simulink model "Model14"  (R2020a)
settings: Solver=VariableStepAuto  StartTime=0.0  StopTime=70  RelTol=1e-3
values from neighbouring files (symbols this model uses):
  Cf = 100000    [Model12_MATscript.m]
  Cr = 110000    [Model12_MATscript.m]
undefined symbols (not defined in the file or in its folder): a, a0, a1, a10, a11, a12, a13, a14, a15, a16, a17, a2, a3, a4, a5, a6, a7, a8, a9, alpha, Area, b, b1, b11, b12, b2, banking_indy, bankingON, C_fuel, camber, curveCenters, Cx, Cz, distanceThreshold, g, init_vel, init_x_pos, init_y_pos, init_yaw, IT, K_wear, l_f, l_r, longStraight, lookahead, m_fuel, mT, overlapThreshold, radius_second_lane, rho_0, rho_1, shortStraight, slipstreamON, trajec, turn, TyreContactAreaFront, TyreContactAreaRear, w1, w2
libraries: simulink x5
(part 1 of 2)
settings Model: PacingRate=2  Creator=carmelo  LastModifiedBy=cvalo

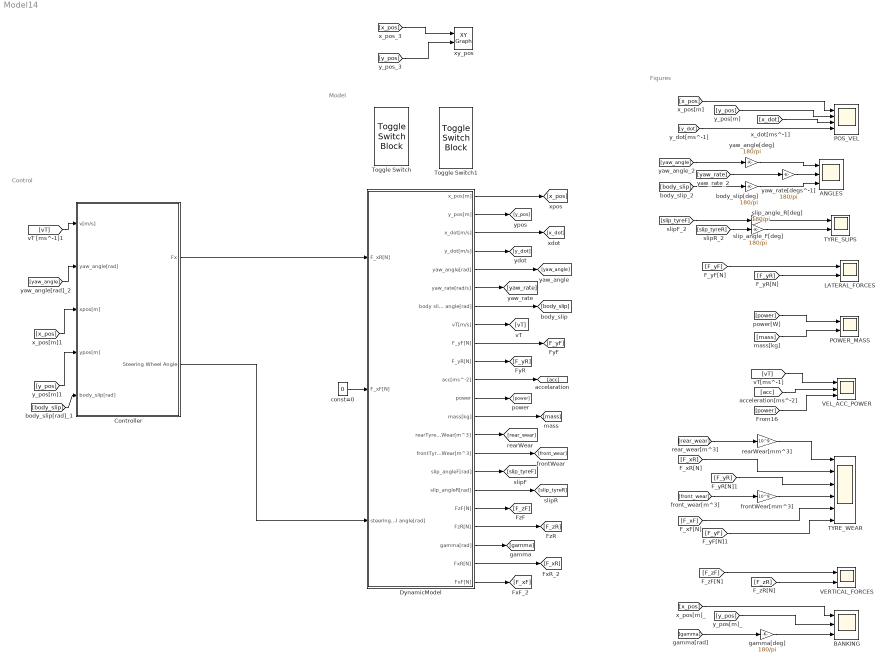
== system Model14 ==
  note: Control
  note: Model
  note: Figures
  ANGLES : Scope  NumInputPorts=3
  BANKING : Scope  NumInputPorts=3
  Controller : Subsystem
  DynamicModel : Subsystem
  LATERAL_FORCES : Scope  NumInputPorts=2
  POS_VEL : Scope  NumInputPorts=4
  POWER_MASS : Scope  NumInputPorts=2
  TYRE_SLIPS : Scope  NumInputPorts=2
  TYRE_WEAR : Scope  NumInputPorts=6
  Toggle Switch : ToggleSwitchBlock
      settings: Values={{'Off', 'On'}, [0 1]}
  Toggle Switch1 : ToggleSwitchBlock
      settings: Values={{'Off', 'On'}, [0 1]}
  VEL_ACC_POWER : Scope  NumInputPorts=3
  VERTICAL_FORCES : Scope  NumInputPorts=2
  body_slip[deg] : Gain  Gain=180/pi
  const=0 : Constant  Value=0
  frontWear[mm^3] : Gain  Gain=10^9
  gamma[deg] : Gain  Gain=180/pi
  rearWear[mm^3] : Gain  Gain=10^9
  slip_angle_F[deg] : Gain  Gain=180/pi
  slip_angle_R[deg] : Gain  Gain=180/pi
  xy_pos : simulink/Sinks/XY Graph  xmin=-900  xmax=900  ymin=-50  ymax=800  st=-1
  yaw_angle[deg] : Gain  Gain=180/pi
  yaw_rate[degs^-1] : Gain  Gain=180/pi
  wires:
  DynamicModel/3(x_dot[m/s]) -> [x_dot]
  DynamicModel/4(y_dot[m/s]) -> [y_dot]
  DynamicModel/1(x_pos[m]) -> [x_pos]
  DynamicModel/2(y_pos[m]) -> [y_pos]
  Controller/2(Steering Wheel Angle) -> DynamicModel/3(steering wheel angle[rad])
  DynamicModel/5(yaw_angle[rad]) -> [yaw_angle]
  DynamicModel/6(yaw_rate[rad/s]) -> [yaw_rate]
  DynamicModel/7(body slip angle[rad]) -> [body_slip]
  DynamicModel/8(vT[m/s]) -> [vT]
  DynamicModel/9(F_yF[N]) -> [F_yF]
  DynamicModel/10(F_yR[N]) -> [F_yR]
  DynamicModel/11(acc[ms^-2]) -> [acc]
  DynamicModel/12(power) -> [power]
  DynamicModel/13(mass[kg]) -> [mass]
  DynamicModel/15(frontTyreWear[m^3]) -> [front_wear]
  DynamicModel/14(rearTyreWear[m^3]) -> [rear_wear]
  DynamicModel/16(slip_angleF[rad]) -> [slip_tyreF]
  DynamicModel/17(slip_angleR[rad]) -> [slip_tyreR]
  slip_angle_R[deg]/1 -> TYRE_SLIPS/2
  [x_pos] -> POS_VEL/1
  [front_wear] -> frontWear[mm^3]/1
  [mass] -> POWER_MASS/2
  yaw_rate[degs^-1]/1 -> ANGLES/2
  body_slip[deg]/1 -> ANGLES/3
  [yaw_angle] -> yaw_angle[deg]/1
  [y_dot] -> POS_VEL/4
  [y_pos] -> POS_VEL/2
  [yaw_rate] -> yaw_rate[degs^-1]/1
  [body_slip] -> body_slip[deg]/1
  [power] -> POWER_MASS/1
  [acc] -> VEL_ACC_POWER/2
  [rear_wear] -> rearWear[mm^3]/1
  yaw_angle[deg]/1 -> ANGLES/1
  [F_yR] -> LATERAL_FORCES/2
  [slip_tyreR] -> slip_angle_R[deg]/1
  [slip_tyreF] -> slip_angle_F[deg]/1
  [F_yF] -> LATERAL_FORCES/1
  [power] -> VEL_ACC_POWER/3
  [x_dot] -> POS_VEL/3
  slip_angle_F[deg]/1 -> TYRE_SLIPS/1
  [vT] -> VEL_ACC_POWER/1
  rearWear[mm^3]/1 -> TYRE_WEAR/1
  frontWear[mm^3]/1 -> TYRE_WEAR/4
  [x_pos] -> xy_pos/1
  [y_pos] -> xy_pos/2
  const=0/1 -> DynamicModel/2(F_xF[N])
  Controller/1(Fx) -> DynamicModel/1(F_xR[N])
  [F_xF] -> TYRE_WEAR/5
  [F_yF] -> TYRE_WEAR/6
  [F_xR] -> TYRE_WEAR/2
  [F_yR] -> TYRE_WEAR/3
  [vT] -> Controller/1(v[m/s])
  DynamicModel/18(FzF[N]) -> [F_zF]
  DynamicModel/19(FzR[N]) -> [F_zR]
  DynamicModel/20(gamma[rad]) -> [gamma]
  [F_zF] -> VERTICAL_FORCES/1
  [F_zR] -> VERTICAL_FORCES/2
  [y_pos] -> BANKING/2
  [x_pos] -> BANKING/1
  [gamma] -> gamma[deg]/1
  gamma[deg]/1 -> BANKING/3
  [yaw_angle] -> Controller/2(yaw_angle[rad])
  [y_pos] -> Controller/4(ypos[m])
  [x_pos] -> Controller/3(xpos[m])
  DynamicModel/21(FxR[N]) -> [F_xR]
  DynamicModel/22(FxF[N]) -> [F_xF]
  [body_slip] -> Controller/5(body_slip[rad])

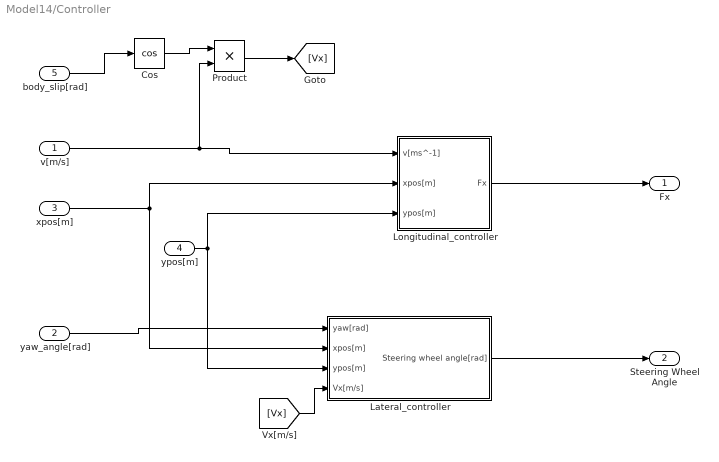
== system Model14/Controller ==
  v[m/s] : Inport  Unit=m/s
  yaw_angle[rad] : Inport  Port=2
  xpos[m] : Inport  Port=3
  ypos[m] : Inport  Port=4
  body_slip[rad] : Inport  Port=5
  Cos : Trigonometry  Operator=cos
  Lateral_controller : Subsystem
  Longitudinal_controller : Subsystem
  Product : Product
  Fx : Outport  Unit=N
  Steering Wheel Angle : Outport  Port=2  Unit=rad
  wires:
  Lateral_controller/1(Steering wheel angle[rad]) -> Steering Wheel Angle/1
  v[m/s]/1 -> Product/2, Longitudinal_controller/1(v[ms^-1])
  yaw_angle[rad]/1 -> Lateral_controller/1(yaw[rad])
  xpos[m]/1 -> Lateral_controller/2(xpos[m]), Longitudinal_controller/2(xpos[m])
  ypos[m]/1 -> Lateral_controller/3(ypos[m]), Longitudinal_controller/3(ypos[m])
  Longitudinal_controller/1(Fx) -> Fx/1
  body_slip[rad]/1 -> Cos/1
  Cos/1 -> Product/1
  Product/1 -> [Vx]
  [Vx] -> Lateral_controller/4(Vx[m/s])

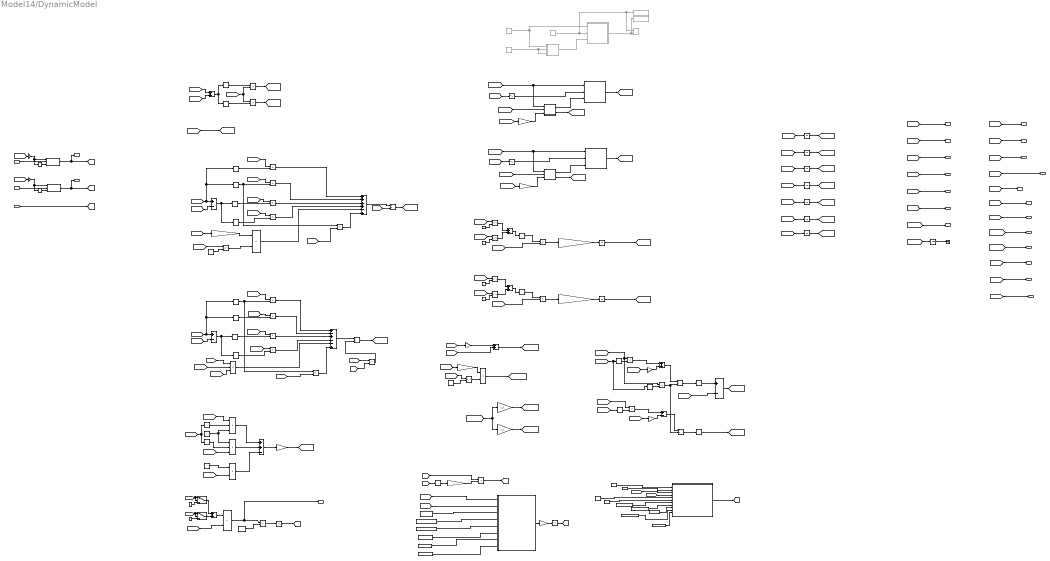
== system Model14/DynamicModel ==
  note: Inputs
  note: Wind effect
  note: FN
  note: Tyre wears
  note: Outputs
  note: Tires slip angles
  note: Tire lateral forces
  note: x6_dot equation
  note: Continuos integration
  note: x4_dot equation
  note: x3_dot equation
  note: x1_dot and x2_dot equations
  note: x5_dot equation
  note: mdot
  note: vertical force
  F_xR[N] : Inport  Unit=N
  F_xF[N] : Inport  Port=2  Unit=N
  steering wheel angle[rad] : Inport  Port=3  Unit=rad
  (F_xR+F_xF)*vT : Product
  (F_xR+F_xF)*vT*c_fuel : Product
  -FxmaxF : UnaryMinus
  -FxmaxR : UnaryMinus
  -b*x6+vT*sin(x5) : Sum  Inputs=+-
  -banking : UnaryMinus
  -slip_angle_F : UnaryMinus
  -slip_angle_R : UnaryMinus
  Banking : MATLAB Function  TreatAsAtomicUnit=on
  BankingON-OFF : Constant  Value=bankingON
  Calculate Peak F : Subsystem
  Calculate Peak F1 : Subsystem  Commented=on
  Calculate Peak R : Subsystem
  Constant : Constant  Value=banking_indy
  FNx*cos(x5) : Product
  FNx*sin(x5) : Product
  FNx_4 : Product
  F_aerod : Product
  F_lift_3 : Product
  F_xF*cos(x5-delta) : Product
  F_xF*sin(x5-delta) : Product
  F_xR*cos(x5) : Product
  F_xR*sin(x5) : Product
  F_xR+F_xF : Sum
  F_yF*cos(x5-delta) : Product
  F_yF*sin(x5-delta) : Product
  F_yR*cos(x5) : Product
  F_yR*sin(x5) : Product
  FrontWearDot : Gain  Gain=K_wear/TyreContactAreaFront
  FrontWearIntegrator : Integrator
  Front_Wear*10^9 : Gain  Gain=10^9
  FxF^2 : Math  Operator=pow  SaturateOnIntegerOverflow=on
  FxF^2+FyF^2 : Sum
  FxR^2 : Math  Operator=pow  SaturateOnIntegerOverflow=on
  FxR^2+FyR^2 : Sum
  FyF^2 : Math  Operator=pow  SaturateOnIntegerOverflow=on
  FyR^2 : Math  Operator=pow  SaturateOnIntegerOverflow=on
  Fz*lf : Gain  Gain=l_f
  Fz*lr : Gain  Gain=l_r
  FzF*sqrt(FxF^2+FyF^2) : Product
  FzR*sqrt(FxR^2+FyR^2) : Product
  PacejkaF : Subsystem
  PacejkaF1 : Subsystem  Commented=on
  PacejkaR : Subsystem
  RearWearDot : Gain  Gain=K_wear/TyreContactAreaRear
  RearWearIntegrator : Integrator
  Rear_Wear*10^9 : Gain  Gain=10^9
  Saturation Dynamic : simulink/Discontinuities/Saturation Dynamic  OutMin=[]  OutMax=[]  OutDataTypeStr=Inherit: Same as second input  OutDataType=fixdt(1, 16)  OutScaling=2^-10  DoSatur=off
  Saturation Dynamic1 : simulink/Discontinuities/Saturation Dynamic  OutMin=[]  OutMax=[]  OutDataTypeStr=Inherit: Same as second input  OutDataType=fixdt(1, 16)  OutScaling=2^-10  DoSatur=off
  Terminator : Terminator
  To Workspace : ToWorkspace  Commented=on  VariableName=alfaPaj  SaveFormat=Timeseries  SampleTime=-1
  To Workspace1 : ToWorkspace  Commented=on  VariableName=FyPaj  SaveFormat=Timeseries  SampleTime=-1
  WindEffect : MATLAB Function  TreatAsAtomicUnit=on
  XY Graph : simulink/Sinks/XY Graph  Commented=on  xmin=-1  xmax=1  ymin=-8500  ymax=8500  st=-1
  a*F_xF*sin(delta) : Product  Inputs=3
  a*F_xF*sin(delta)+ a*F_yF*cos(delta)+ b*F_yR : Sum  Inputs=++-
  a*F_yF*cos(delta) : Product  Inputs=3
  a*x6 : Gain  Gain=a
  a*x6+vT*sin(x5) : Sum
  a*x6+vT*sin(x5) -------------------- vT*cos(x5) : Product  Inputs=*/
  alpha : Constant  Value=alpha
  alpha-1+1 : simulink/Sources/Ramp  Commented=on  slope=0.02  start=0  InitialOutput=-1
  atan(-b*x6+vT*sin(x5) -------------------- vT*cos(x5)) : Trigonometry  Operator=atan
  atan(a*x6+vT*sin(x5) -------------------- vT*cos(x5)) : Trigonometry  Operator=atan
  b*F_yR : Product
  b*x6 : Gain  Gain=b
  b*x6+vT*sin(x5) -------------------- vT*cos(x5) : Product  Inputs=*/
  bankingAngle : Constant  Value=turn
  bankingThreshL : Constant  Value=longStraight
  bankingThreshS : Constant  Value=shortStraight
  bankingToRad : Gain  Gain=pi/180
  c_fuel : Constant  Value=C_fuel
  const=-5.625 : Constant  Value=-5.625
  const=0 : Constant  Value=0
  const=0_2 : Constant  Value=0
  const=0_5 : Constant  Commented=on  Value=0
  const=10 : Constant  Value=10
  const=2 : Constant  Value=2
  const=2_{2..6} (5 alike) : Constant  Value=2
  const=Fz : Constant  Commented=on  Value=4000
  const=a : Constant  Value=a
  const=b : Constant  Value=b
  const=g : Gain  Gain=g
  cos(delta)_2 : Trigonometry  Operator=cos
  cos(x3+x5) : Trigonometry  Operator=cos
  cos(x5) : Trigonometry  Operator=cos
  cos(x5)_2 : Trigonometry  Operator=cos
  cos(x5)_3 : Trigonometry  Operator=cos
  cos(x5-delta) : Trigonometry  Operator=cos
  cos(x5-delta)_2 : Trigonometry  Operator=cos
  curveCenters : Constant  Value=curveCenters
  curveCenters_2 : Constant  Value=curveCenters
  dTresh : Constant  Value=distanceThreshold
  eps : Gain  Gain=0.99999
  eps_2 : Gain  Gain=0.99999
  g*sin(gamma) : Gain  Gain=g
  mT*vT : Product
  mT*vt*x6 : Product  Inputs=3
  mT+F_lift : Sum
  mTdot_2 : UnaryMinus
  mTintegrator : Integrator  InitialCondition=mT  LimitOutput=on  UpperSaturationLimit=mT  LowerSaturationLimit=mT - m_fuel
  oTresh : Constant  Value=overlapThreshold
  rho*area*Cz*0.5 : Gain  Gain=Area*Cz*0.5
  rho*area*cx*0.5 : Gain  Gain=Area*Cx*0.5
  rho_0 : Constant  Value=rho_0
  rho_1 : Constant  Value=rho_1
  sin(delta)_2 : Trigonometry
  sin(gamma) : Trigonometry
  sin(x3+x5) : Trigonometry
  sin(x5) : Trigonometry
  sin(x5)_2 : Trigonometry
  sin(x5)_3 : Trigonometry
  sin(x5)_4 : Trigonometry
  sin(x5-delta) : Trigonometry
  sin(x5-delta)_2 : Trigonometry
  slip_angle_F_3 : Sum  Inputs=+-
  slipstreamON-OFF : Constant  Value=slipstreamON
  sqrt(FxF^2+FyF^2) : Sqrt  SaturateOnIntegerOverflow=on
  sqrt(FxR^2+FyR^2) : Sqrt  SaturateOnIntegerOverflow=on
  switch_FxF-0 : Switch
  switch_FxR-0 : Switch
  v2pos : Integrator  LimitOutput=on  LowerSaturationLimit=0
  vT*cos(x3+x5) : Product
  vT*cos(x5)_2 : Product
  vT*sin(x3+x5) : Product
  vT*sin(x5)_2 : Product
  vT*sin(x5)_3 : Product
  vT^2 : Math  Operator=pow  SaturateOnIntegerOverflow=on
  vT^2_2 : Math  Operator=pow  SaturateOnIntegerOverflow=on
  x1integrator : Integrator  InitialCondition=init_x_pos
  x2integrator : Integrator  InitialCondition=init_y_pos
  x3+x5 : Sum
  x3integrator : Integrator  InitialCondition=init_yaw
  x4dot*mT : Sum  Inputs=++++-+
  x4dot_2 : Product  Inputs=*/
  x4integrator : Integrator  InitialCondition=init_vel  LimitOutput=on  UpperSaturationLimit=76  LowerSaturationLimit=0
  x5-delta : Sum  Inputs=+-
  x5-delta_2 : Sum  Inputs=+-
  x5dot*mT*x4 : Sum  Inputs=+-+--+
  x5dot_2 : Product  Inputs=*/
  x5integrator : Integrator
  x6_dot_2 : Gain  Gain=1/IT
  x6integrator : Integrator
  x_pos[m] : Outport  Unit=m
  y_pos[m] : Outport  Port=2  Unit=m
  x_dot[m/s] : Outport  Port=3  Unit=m/s
  y_dot[m/s] : Outport  Port=4  Unit=m/s
  yaw_angle[rad] : Outport  Port=5  Unit=rad
  yaw_rate[rad/s] : Outport  Port=6  Unit=rad/s
  body slip angle[rad] : Outport  Port=7  Unit=rad
  vT[m/s] : Outport  Port=8  Unit=m/s
  F_yF[N] : Outport  Port=9  Unit=N
  F_yR[N] : Outport  Port=10  Unit=N
  acc[ms^-2] : Outport  Port=11  Unit=m/s^2
  power : Outport  Port=12  Unit=watt
  mass[kg] : Outport  Port=13  Unit=kg
  rearTyreWear[m^3] : Outport  Port=14  Unit=m^3
  frontTyreWear[m^3] : Outport  Port=15  Unit=m^3
  slip_angleF[rad] : Outport  Port=16  Unit=rad
  slip_angleR[rad] : Outport  Port=17  Unit=rad
  FzF[N] : Outport  Port=18  Unit=N
  FzR[N] : Outport  Port=19  Unit=N
  gamma[rad] : Outport  Port=20  Unit=rad
  FxR[N] : Outport  Port=21  Unit=N
  FxF[N] : Outport  Port=22  Unit=N
  wires:
  [x5_slip_angle] -> sin(x5)_4/1
  [x4_vT] -> vT*sin(x5)_3/1
  atan(a*x6+vT*sin(x5) -------------------- vT*cos(x5))/1 -> slip_angle_F_3/1
  [x1_x_pos] -> x_pos[m]/1
  [x6_yaw_rate] -> a*x6/1
  [F_yR] -> b*F_yR/2
  sin(x3+x5)/1 -> vT*sin(x3+x5)/2
  x4integrator/1 -> [x4_vT]
  sin(x5)/1 -> F_yR*sin(x5)/2, FNx*sin(x5)/1
  F_yR*sin(x5)/1 -> x4dot*mT/2
  [x3_dot] -> x3integrator/1
  b*x6+vT*sin(x5) -------------------- vT*cos(x5)/1 -> atan(-b*x6+vT*sin(x5) -------------------- vT*cos(x5))/1
  F_xF*cos(x5-delta)/1 -> x4dot*mT/3
  [F_yF] -> F_yF*cos(x5-delta)/1
  vT*cos(x5)_2/1 -> a*x6+vT*sin(x5) -------------------- vT*cos(x5)/2, b*x6+vT*sin(x5) -------------------- vT*cos(x5)/2
  [x5_slip_angle] -> sin(x5)/1, cos(x5)/1, x5-delta/1
  slip_angle_F_3/1 -> [slip_angle_F]
  cos(x5)/1 -> F_xR*cos(x5)/2
  [x5_slip_angle] -> x3+x5/2
  sin(x5)_4/1 -> vT*sin(x5)_3/2
  x6integrator/1 -> [x6_yaw_rate]
  [x4_dot] -> x4integrator/1
  vT*cos(x3+x5)/1 -> [x1_dot]
  [x3_yaw_angle] -> yaw_angle[rad]/1
  [x1_dot] -> x_dot[m/s]/1
  const=b/1 -> b*F_yR/1
  cos(x5-delta)_2/1 -> F_yF*cos(x5-delta)/2
  [x2_dot] -> x2integrator/1
  x5-delta/1 -> sin(x5-delta)/1, cos(x5-delta)/1
  [x6_dot] -> x6integrator/1
  x3integrator/1 -> [x3_yaw_angle]
  a*x6/1 -> a*x6+vT*sin(x5)/2
  [x2_y_pos] -> y_pos[m]/1
  cos(x5-delta)/1 -> F_xF*cos(x5-delta)/2
  x6_dot_2/1 -> [x6_dot]
  [x4_vT] -> mT*vt*x6/2
  [x6_yaw_rate] -> [x3_dot]
  [F_yF] -> F_yF*sin(x5-delta)/1
  [x3_yaw_angle] -> x3+x5/1
  [x6_yaw_rate] -> yaw_rate[rad/s]/1
  [F_yR] -> F_yR*sin(x5)/1
  [x4_vT] -> vT[m/s]/1
  a*F_xF*sin(delta)/1 -> a*F_xF*sin(delta)+ a*F_yF*cos(delta)+ b*F_yR/1
  [F_yR] -> F_yR*cos(x5)/1
  atan(-b*x6+vT*sin(x5) -------------------- vT*cos(x5))/1 -> [slip_angle_R]
  a*x6+vT*sin(x5) -------------------- vT*cos(x5)/1 -> atan(a*x6+vT*sin(x5) -------------------- vT*cos(x5))/1
  [x4_vT] -> vT*sin(x3+x5)/1, vT*cos(x3+x5)/2
  vT*sin(x3+x5)/1 -> [x2_dot]
  cos(x5)_2/1 -> F_yR*cos(x5)/2, FNx*cos(x5)/1
  sin(delta)_2/1 -> a*F_xF*sin(delta)/2
  -b*x6+vT*sin(x5)/1 -> b*x6+vT*sin(x5) -------------------- vT*cos(x5)/1
  [x5_slip_angle] -> cos(x5)_3/1, sin(x5)_3/1
  sin(x5)_2/1 -> F_xR*sin(x5)/2
  [x6_yaw_rate] -> mT*vt*x6/3
  cos(delta)_2/1 -> a*F_yF*cos(delta)/2
  a*F_xF*sin(delta)+ a*F_yF*cos(delta)+ b*F_yR/1 -> x6_dot_2/1
  cos(x3+x5)/1 -> vT*cos(x3+x5)/1
  b*F_yR/1 -> a*F_xF*sin(delta)+ a*F_yF*cos(delta)+ b*F_yR/3
  cos(x5)_3/1 -> vT*cos(x5)_2/2
  x1integrator/1 -> [x1_x_pos]
  x3+x5/1 -> cos(x3+x5)/1, sin(x3+x5)/1
  a*F_yF*cos(delta)/1 -> a*F_xF*sin(delta)+ a*F_yF*cos(delta)+ b*F_yR/2
  F_yF*sin(x5-delta)/1 -> x4dot*mT/4
  steering wheel angle[rad]/1 -> [delta]
  vT*sin(x5)_2/1 -> a*x6+vT*sin(x5)/1
  [x5_dot] -> x5integrator/1
  F_xF*sin(x5-delta)/1 -> x5dot*mT*x4/4
  vT*sin(x5)_3/1 -> -b*x6+vT*sin(x5)/1
  [x4_vT] -> vT*sin(x5)_2/1, vT*cos(x5)_2/1
  [mT] -> mT*vt*x6/1
  sin(x5-delta)_2/1 -> F_xF*sin(x5-delta)/2
  x5dot*mT*x4/1 -> x5dot_2/1
  F_yF*cos(x5-delta)/1 -> x5dot*mT*x4/3
  [x5_slip_angle] -> sin(x5)_2/1, cos(x5)_2/1, x5-delta_2/1
  const=a/1 -> a*F_xF*sin(delta)/3, a*F_yF*cos(delta)/1
  x5dot_2/1 -> [x5_dot]
  x2integrator/1 -> [x2_y_pos]
  [F_yF] -> a*F_yF*cos(delta)/3
  x5-delta_2/1 -> sin(x5-delta)_2/1, cos(x5-delta)_2/1
  mT*vt*x6/1 -> x5dot*mT*x4/5
  F_yR*cos(x5)/1 -> x5dot*mT*x4/1
  sin(x5-delta)/1 -> F_yF*sin(x5-delta)/2
  [x6_yaw_rate] -> b*x6/1
  [x1_dot] -> x1integrator/1
  [x2_dot] -> y_dot[m/s]/1
  F_xR*cos(x5)/1 -> x4dot*mT/1
  sin(x5)_3/1 -> vT*sin(x5)_2/2
  x5integrator/1 -> [x5_slip_angle]
  F_xR*sin(x5)/1 -> x5dot*mT*x4/2
  a*x6+vT*sin(x5)/1 -> a*x6+vT*sin(x5) -------------------- vT*cos(x5)/1
  b*x6/1 -> -b*x6+vT*sin(x5)/2
  x4dot_2/1 -> [x4_dot]
  x4dot*mT/1 -> x4dot_2/1
  [F_yF] -> F_yF[N]/1
  [F_yR] -> F_yR[N]/1
  [x5_slip_angle] -> body slip angle[rad]/1
  [x4_dot] -> acc[ms^-2]/1
  mT*vT/1 -> x5dot_2/2
  [mT] -> mT*vT/1
  [x4_vT] -> vT^2/1
  F_aerod/1 -> x4dot*mT/5
  [rho] -> rho*area*cx*0.5/1
  const=2/1 -> vT^2/2
  rho*area*cx*0.5/1 -> F_aerod/1
  vT^2/1 -> F_aerod/2
  (F_xR+F_xF)*vT/1 -> (F_xR+F_xF)*vT*c_fuel/1, power/1
  F_xR+F_xF/1 -> (F_xR+F_xF)*vT/1
  c_fuel/1 -> (F_xR+F_xF)*vT*c_fuel/2
  [x4_vT] -> (F_xR+F_xF)*vT/2
  mT+F_lift/1 -> [F_z]
  [F_lift] -> mT+F_lift/2
  [mT] -> const=g/1
  (F_xR+F_xF)*vT*c_fuel/1 -> mTdot_2/1
  mTdot_2/1 -> [mTdot]
  [mTdot] -> mTintegrator/1
  mTintegrator/1 -> [mT]
  [mT] -> mass[kg]/1
  [mT] -> x4dot_2/2
  [F_zR] -> FzR*sqrt(FxR^2+FyR^2)/2
  FzR*sqrt(FxR^2+FyR^2)/1 -> RearWearDot/1
  RearWearDot/1 -> RearWearIntegrator/1
  RearWearIntegrator/1 -> [RearWear]
  [RearWear] -> rearTyreWear[m^3]/1
  [FrontWear] -> frontTyreWear[m^3]/1
  FrontWearIntegrator/1 -> [FrontWear]
  [FNX] -> FNx*sin(x5)/2
  FNx*sin(x5)/1 -> x4dot*mT/6
  [FNX] -> FNx*cos(x5)/2
  FNx*cos(x5)/1 -> x5dot*mT*x4/6
  sin(gamma)/1 -> g*sin(gamma)/1
  [gamma] -> sin(gamma)/1
  vT^2_2/1 -> F_lift_3/2
  rho*area*Cz*0.5/1 -> F_lift_3/1
  const=2_6/1 -> vT^2_2/2
  [x4_vT] -> vT^2_2/1
  [rho] -> rho*area*Cz*0.5/1
  F_lift_3/1 -> [F_lift]
  [x1_x_pos] -> Banking/1(x)
  [x2_y_pos] -> Banking/2(y)
  curveCenters/1 -> Banking/3(curveCenters)
  bankingAngle/1 -> Banking/6(curve)
  Fz*lf/1 -> [F_zF]
  [F_z] -> Fz*lr/1, Fz*lf/1
  Fz*lr/1 -> [F_zR]
  g*sin(gamma)/1 -> FNx_4/2
  const=0/1 -> switch_FxR-0/3
  switch_FxR-0/1 -> F_xR+F_xF/1
  switch_FxF-0/1 -> F_xR+F_xF/2
  const=0_2/1 -> switch_FxF-0/3
  sqrt(FxR^2+FyR^2)/1 -> FzR*sqrt(FxR^2+FyR^2)/1
  FxR^2+FyR^2/1 -> sqrt(FxR^2+FyR^2)/1
  [F_xR] -> FxR^2/1
  const=2_2/1 -> FxR^2/2
  [F_yR] -> FyR^2/1
  const=2_3/1 -> FyR^2/2
  FyR^2/1 -> FxR^2+FyR^2/2
  FxR^2/1 -> FxR^2+FyR^2/1
  [F_zF] -> FzF*sqrt(FxF^2+FyF^2)/2
  [F_xF] -> FxF^2/1
  FzF*sqrt(FxF^2+FyF^2)/1 -> FrontWearDot/1
  FxF^2+FyF^2/1 -> sqrt(FxF^2+FyF^2)/1
  [F_yF] -> FyF^2/1
  FxF^2/1 -> FxF^2+FyF^2/1
  FyF^2/1 -> FxF^2+FyF^2/2
  const=2_4/1 -> FxF^2/2
  FrontWearDot/1 -> FrontWearIntegrator/1
  const=2_5/1 -> FyF^2/2
  sqrt(FxF^2+FyF^2)/1 -> FzF*sqrt(FxF^2+FyF^2)/1
  const=g/1 -> mT+F_lift/1
  [mT] -> FNx_4/1
  FNx_4/1 -> [FNX]
  PacejkaR/1(Fy) -> [F_yR]
  PacejkaF/1(Fy) -> [F_yF]
  [slip_angle_R] -> -slip_angle_R/1
  -slip_angle_R/1 -> PacejkaR/2(slip[rad])
  [slip_angle_F] -> -slip_angle_F/1
  -slip_angle_F/1 -> PacejkaF/2(slip[rad])
  [F_zF] -> Calculate Peak F/1(Fz), PacejkaF/1(Fz[N])
  Calculate Peak F/1(Peak) -> PacejkaF/3(D)
  [F_xF] -> Calculate Peak F/2(Fx)
  [FrontWear] -> Front_Wear*10^9/1
  Front_Wear*10^9/1 -> Calculate Peak F/3(Wear)
  [RearWear] -> Rear_Wear*10^9/1
  [F_xR] -> Calculate Peak R/2(Fx)
  [F_zR] -> PacejkaR/1(Fz[N]), Calculate Peak R/1(Fz)
  Calculate Peak R/1(Peak) -> PacejkaR/3(D)
  Rear_Wear*10^9/1 -> Calculate Peak R/3(Wear)
  rho_0/1 -> WindEffect/1(rho_0)
  rho_1/1 -> WindEffect/2(rho_1)
  [x2_y_pos] -> WindEffect/4(ego_y)
  [x1_x_pos] -> WindEffect/3(ego_x)
  [slip_angle_F] -> slip_angleF[rad]/1
  [slip_angle_R] -> slip_angleR[rad]/1
  const=10/1 -> WindEffect/5(opp_x)
  const=-5.625/1 -> WindEffect/6(opp_y)
  dTresh/1 -> WindEffect/7(distanceThreshold)
  oTresh/1 -> WindEffect/8(overlapThreshold)
  alpha/1 -> WindEffect/9(alpha)
  curveCenters_2/1 -> WindEffect/10(curveCenters)
  bankingThreshL/1 -> Banking/4(longStraight)
  bankingThreshS/1 -> Banking/5(shortStraight)
  WindEffect/1(aerodynamic_coeff) -> [rho]
  Banking/1(res) -> bankingToRad/1
  [F_xR] -> F_xR*cos(x5)/1
  [F_xR] -> F_xR*sin(x5)/1
  [F_xR] -> switch_FxR-0/2, switch_FxR-0/1
  [F_xF] -> switch_FxF-0/2, switch_FxF-0/1
  [F_xF] -> F_xF*cos(x5-delta)/1
  [F_xF] -> F_xF*sin(x5-delta)/1
  [F_xF] -> a*F_xF*sin(delta)/1
  [delta] -> x5-delta/2
  [delta] -> x5-delta_2/2
  [delta] -> cos(delta)_2/1, sin(delta)_2/1
  [delta] -> slip_angle_F_3/2
  [x4_vT] -> mT*vT/2
  Calculate Peak F1/1(Peak) -> PacejkaF1/3(D)
  const=0_5/1 -> Calculate Peak F1/3(Wear), Calculate Peak F1/2(Fx)
  const=Fz/1 -> Calculate Peak F1/1(Fz), PacejkaF1/1(Fz[N])
  PacejkaF1/1(Fy) -> To Workspace1/1, XY Graph/2
  alpha-1+1/1 -> XY Graph/1, To Workspace/1, PacejkaF1/2(slip[rad])
  slipstreamON-OFF/1 -> WindEffect/11(slipstreamON)
  BankingON-OFF/1 -> Banking/7(bankingON)
  -banking/1 -> [gamma]
  bankingToRad/1 -> -banking/1
  Constant/1 -> Banking/8(banking_indy)
  Calculate Peak F/2(Fxmax) -> [F_xmaxF]
  Calculate Peak R/2(Fxmax) -> [F_xmaxR]
  F_xR[N]/1 -> Saturation Dynamic/2
  Saturation Dynamic/1 -> FxR[N]/1, [F_xR]
  [F_xmaxR] -> eps/1
  -FxmaxR/1 -> Saturation Dynamic/3
  F_xF[N]/1 -> Saturation Dynamic1/2
  Saturation Dynamic1/1 -> FxF[N]/1, [F_xF]
  [F_xmaxF] -> eps_2/1
  -FxmaxF/1 -> Saturation Dynamic1/3
  [F_zR] -> FzR[N]/1
  [F_zF] -> FzF[N]/1
  [gamma] -> gamma[rad]/1
  [x4_vT] -> v2pos/1
  v2pos/1 -> Terminator/1
  eps/1 -> Saturation Dynamic/1, -FxmaxR/1
  eps_2/1 -> Saturation Dynamic1/1, -FxmaxF/1

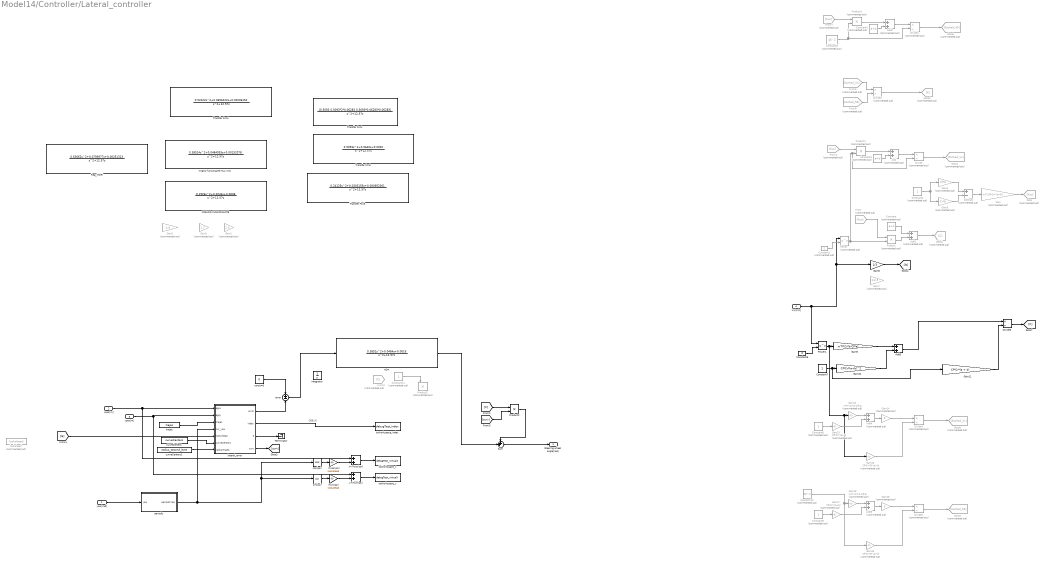
== system Model14/Controller/Lateral_controller ==
  note: DEBUG
  yaw[rad] : Inport
  xpos[m] : Inport  Port=2
  ypos[m] : Inport  Port=3
  Vx[m/s] : Inport  Port=4
  Add{,1..2,4..5} (5 alike) : Sum  Commented=on
  Add3 : Sum
  Constant : Constant  Commented=on  Value=a+b
  Constant1 : Constant  Commented=on  Value=2
  Constant10 : Constant  Commented=on  Value=50^2
  Constant{2,8..9,11} (4 alike) : Constant  Commented=on
  Constant3 : Constant  Commented=on  Value=a+b
  Constant4 : Constant  Commented=on  Value=a+b
  Constant5 : Constant  Commented=on  Value=45^2
  Constant6 : Constant  Value=2
  Constant7 : Constant
  Divide{,1..2,4..5} (5 alike) : Product  Commented=on  Inputs=*/
  Divide3 : Product  Inputs=*/
  From : From  Commented=on  GotoTag=Kus
  From1 : From  Commented=on  GotoTag=Kus
  From5 : From  Commented=on  GotoTag=K
  From6 : From  Commented=on  GotoTag=Ksched_Vx
  From7 : From  Commented=on  GotoTag=Kus
  From8 : From  Commented=on  GotoTag=Ksched_50
  Gain : Gain  Commented=on  Gain=mT/(Cf*Cr*(a+b))
  Gain1 : Gain  Commented=on  Gain=2.5
  Gain10 : Gain  Gain=Cf*Cr*(a+b)^2
  Gain11 : Gain  Gain=Cf*Cr*(a + b)
  Gain12 : Gain  Commented=on  Gain=mT*(Cr*b-Cf*a)
  Gain13 : Gain  Commented=on  Gain=Cf*Cr*(a+b)
  Gain14 : Gain  Commented=on  Gain=3
  Gain15 : Gain  Commented=on  Gain=Cf*Cr*3*(a+b)
  Gain16 : Gain  Commented=on  Gain=mT*(Cr*b-Cf*a)
  Gain17 : Gain  Commented=on  Gain=Cf*Cr*(a+b)
  Gain18 : Gain  Commented=on  Gain=3
  Gain19 : Gain  Commented=on  Gain=Cf*Cr*3*(a+b)
  Gain2 : Gain  Commented=on  Gain=0.9
  Gain3 : Gain  Commented=on  Gain=1.7
  Gain4 : Gain  Commented=on  Gain=Cf*a
  Gain5 : Gain  Commented=on  Gain=Cr*b
  Gain6 : Gain  Gain=1/3
  Gain7 : Gain  Commented=on  Gain=1/3.5
  Gain9 : Gain  Gain=mT*(Cr*b-Cf*a)
  Goto : Goto  Commented=on  GotoTag=Kus
  Goto1 : Goto  Commented=on  GotoTag=Ksched_Vx
  Goto2 : Goto  Commented=on  GotoTag=C
  Goto5 : Goto  Commented=on  GotoTag=K
  Goto6 : Goto  Commented=on  GotoTag=Ksched_45
  Goto8 : Goto  Commented=on  GotoTag=Ksched_Vx
  Goto9 : Goto  Commented=on  GotoTag=Ksched_50
  Integrator : Integrator
  MIGLIOR FUNZIONANTE : TransferFcn  Numerator=[0.1926 0.0242 0.0008]  Denominator=[1 12.57 0]
  Power : Math  Commented=on  Operator=pow  SaturateOnIntegerOverflow=on
  Power1 : Math  Operator=pow  SaturateOnIntegerOverflow=on
  Product{,1,3..4} (4 alike) : Product  Commented=on
  Product2 : Product
  Reg_MORI : TransferFcn  Numerator=[0.63662 0.0799977 0.00251313]  Denominator=[1 12.57 0]
  Subtract : Sum  Commented=on  Inputs=+-
  Sum : Sum  Inputs=++|
  Terminator : Terminator
  Transfer Fcn1 : TransferFcn  Numerator=[0.5093 0.5093*2*0.06283 0.5093*0.06283*0.06283]  Denominator=[1 12.57 0]
  Transfer Fcn2 : TransferFcn  Numerator=[0.5093 0.0640 0.0020]  Denominator=[1 12.57 0]
  Transfer Fcn3 : TransferFcn  Numerator=[0.24125 0.0303155 0.000952361]  Denominator=[1 12.57 0]
  Transfer Fcn4 : TransferFcn  Numerator=[0.52222 0.0656222 0.00206152]  Denominator=[1 12.57 0]
  const=0 : Constant  Value=0
  cos(psi) : Trigonometry  Operator=cos
  curveCenters : Constant  Value=curveCenters
  curveCenters1 : Constant  Value=radius_second_lane
  e1m : TransferFcn  Numerator=[0.3852 0.0484 0.0016]  Denominator=[1 12.57 0]
  error : Sum  Inputs=+-
  l*cos(psi) : Gain  Gain=lookahead
  l*sin(psi) : Gain  Gain=lookahead
  lateral_error : MATLAB Function  TreatAsAtomicUnit=on
  lookahead : Constant  Commented=on  Value=lookahead
  miglior funzionante ma x 0.5 : TransferFcn  Numerator=[0.38524 0.0484093 0.00152078]  Denominator=[1 12.57 0]
  periodic : MATLAB Function  TreatAsAtomicUnit=on
  sin(psi) : Trigonometry
  toWorkspace_index : ToWorkspace  VariableName=debugTest_index  SaveFormat=Timeseries  SampleTime=-1
  toWorkspace_x : ToWorkspace  VariableName=debugTest_virtualX  SaveFormat=Timeseries  SampleTime=-1
  toWorkspace_y : ToWorkspace  VariableName=debugTest_virtualY  SaveFormat=Timeseries  SampleTime=-1
  trajec : Constant  Value=trajec
  x+l*cos(psi) : Sum
  y+l*sin(psi) : Sum
  Steering wheel angle[rad] : Outport
  wires:
  yaw[rad]/1 -> periodic/1(yaw)
  periodic/1(periodicYaw) -> sin(psi)/1, cos(psi)/1, lateral_error/4(cur_yaw)
  trajec/1 -> lateral_error/3(trajec)
  xpos[m]/1 -> x+l*cos(psi)/1, lateral_error/1(egox)
  ypos[m]/1 -> y+l*sin(psi)/1, lateral_error/2(egoy)
  lateral_error/1(error) -> error/2
  const=0/1 -> error/1
  lateral_error/2(index) -> toWorkspace_index/1
  cos(psi)/1 -> l*cos(psi)/1
  l*cos(psi)/1 -> x+l*cos(psi)/2
  x+l*cos(psi)/1 -> toWorkspace_x/1
  sin(psi)/1 -> l*sin(psi)/1
  l*sin(psi)/1 -> y+l*sin(psi)/2
  y+l*sin(psi)/1 -> toWorkspace_y/1
  error/1 -> e1m/1
  lateral_error/3(e) -> Terminator/1
  Sum/1 -> Steering wheel angle[rad]/1
  Vx[m/s]/1 -> Power/1, Gain6/1, Power1/1
  Constant1/1 -> Power/2
  Power/1 -> Divide/2, Product1/2, Product/2
  From/1 -> Product/1
  Gain/1 -> Goto/1
  Subtract/1 -> Gain/1
  Constant2/1 -> Gain5/1, Gain4/1
  Gain4/1 -> Subtract/1
  Gain5/1 -> Subtract/2
  Divide/1 -> Goto1/1
  From1/1 -> Product1/1
  Product1/1 -> Add/1
  Constant3/1 -> Add/2
  Add/1 -> Divide/1
  Constant/1 -> Add1/1
  Product/1 -> Add1/2
  Add1/1 -> Goto2/1
  [C] -> Product2/1
  [curv] -> Product2/2
  Product2/1 -> Sum/1
  lateral_error/4(curv) -> [curv]
  Gain6/1 -> [la]
  [la] -> lateral_error/5(lookAhead)
  e1m/1 -> Sum/2
  Divide2/1 -> Goto5/1
  Add2/1 -> Divide1/1
  Divide1/1 -> Goto6/1
  From7/1 -> Product4/1
  Constant5/1 -> Product4/2, Divide1/2
  Product4/1 -> Add2/1
  Constant4/1 -> Add2/2
  From6/1 -> Divide2/1
  From8/1 -> Divide2/2
  curveCenters/1 -> lateral_error/6(curveCenters)
  curveCenters1/1 -> lateral_error/7(radiusTrajec)
  Constant6/1 -> Power1/2
  Power1/1 -> Gain15/1, Gain12/1, Gain9/1
  Gain9/1 -> Add3/1
  Constant7/1 -> Gain11/1, Gain10/1
  Gain10/1 -> Add3/2
  Add3/1 -> Divide3/1
  Divide3/1 -> [C]
  Gain11/1 -> Divide3/2
  Gain12/1 -> Add4/1
  Constant8/1 -> Gain13/1
  Gain13/1 -> Add4/2
  Add4/1 -> Gain14/1
  Gain14/1 -> Divide4/1
  Gain15/1 -> Divide4/2
  Divide4/1 -> Goto8/1
  Gain17/1 -> Add5/2
  Gain19/1 -> Divide5/2
  Constant9/1 -> Gain17/1
  Constant10/1 -> Gain19/1, Gain16/1
  Divide5/1 -> Goto9/1
  Add5/1 -> Gain18/1
  Gain16/1 -> Add5/1
  Gain18/1 -> Divide5/1
  Constant11/1 -> Product3/1

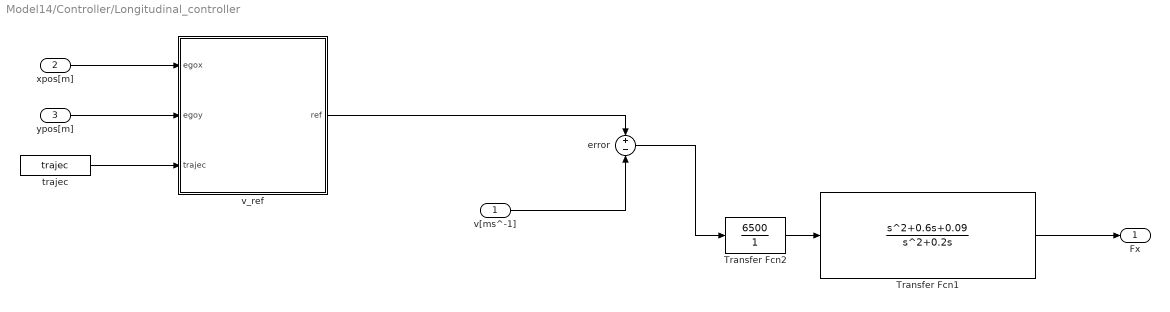
== system Model14/Controller/Longitudinal_controller ==
  v[ms^-1] : Inport
  xpos[m] : Inport  Port=2
  ypos[m] : Inport  Port=3
  Transfer Fcn1 : TransferFcn  Numerator=[1 0.6 0.09]  Denominator=[1 0.2 0]
  Transfer Fcn2 : TransferFcn  Numerator=[6500]  Denominator=[1]
  error : Sum  Inputs=+-
  trajec : Constant  Value=trajec
  v_ref : MATLAB Function  TreatAsAtomicUnit=on
  Fx : Outport
  wires:
  v[ms^-1]/1 -> error/2
  error/1 -> Transfer Fcn2/1
  xpos[m]/1 -> v_ref/1(egox)
  ypos[m]/1 -> v_ref/2(egoy)
  trajec/1 -> v_ref/3(trajec)
  Transfer Fcn2/1 -> Transfer Fcn1/1
  Transfer Fcn1/1 -> Fx/1
  v_ref/1(ref) -> error/1

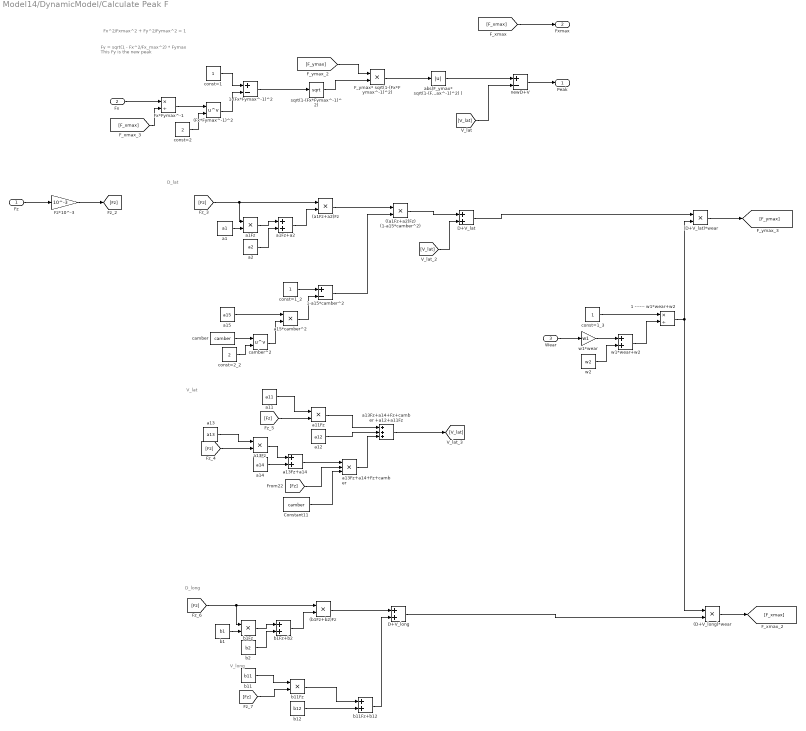
== system Model14/DynamicModel/Calculate Peak F ==
  note: V_lat
  note: D_lat
  note: D_long
  note: V_long
  note: Fy = sqrt(1 - Fx^2/Fx_max^2) * Fymax
      |
      | This Fy is the new peak
  note: Fx^2/Fxmax^2 + Fy^2/Fymax^2 = 1
  Fz : Inport  Unit=N
  Fx : Inport  Port=2  Unit=N
  Wear : Inport  Port=3
  ((a1Fz+a2)Fz) (1-a15*camber^2) : Product
  (D+V_lat)*wear : Product
  (D+V_long)*wear : Product
  (Fx*Fymax^-1)^2 : Math  Operator=pow  SaturateOnIntegerOverflow=on
  (a1Fz+a2)Fz : Product
  (b1Fz+b2)Fz : Product
  1 ------ w1*wear+w2 : Product  Inputs=*/
  1-(Fx*Fymax^-1)^2 : Sum  Inputs=+-
  1-a15*camber^2 : Sum  Inputs=+-
  Constant11 : Constant  Value=camber
  D+V_lat : Sum
  D+V_long : Sum
  "F_ymax* sqrt(1-(Fx*Fymax^-1)^2) " : Product
  Fx*Fymax^-1 : Product  Inputs=*/
  Fz*10^-3 : Gain  Gain=10^-3
  a1 : Constant  Value=a1
  a11 : Constant  Value=a11
  a11Fz : Product
  a12 : Constant  Value=a12
  a13 : Constant  Value=a13
  a13Fz : Product
  a13Fz+a14 : Sum
  a13Fz+a14+Fz+camber : Product  Inputs=3
  a13Fz+a14+Fz+camber +a12+a11Fz : Sum  Inputs=+++
  a14 : Constant  Value=a14
  a15 : Constant  Value=a15
  a15*camber^2 : Product
  a1Fz : Product
  a1Fz+a2 : Sum
  a2 : Constant  Value=a2
  abs(F_ymax* sqrt(1-(Fx*Fymax^-1)^2) ) : Abs
  b1 : Constant  Value=b1
  b11 : Constant  Value=b11
  b11Fz : Product
  b11Fz+b12 : Sum
  b12 : Constant  Value=b12
  b1Fz : Product
  b1Fz+b2 : Sum
  b2 : Constant  Value=b2
  camber : Constant  Value=camber
  camber^2 : Math  Operator=pow  SaturateOnIntegerOverflow=on
  const=1 : Constant
  const=1_2 : Constant
  const=1_3 : Constant
  const=2 : Constant  Value=2
  const=2_2 : Constant  Value=2
  newD+V : Sum  Inputs=+-
  sqrt(1-(Fx*Fymax^-1)^2) : Sqrt  SaturateOnIntegerOverflow=on
  w1*wear : Gain  Gain=w1
  w1*wear+w2 : Sum
  w2 : Constant  Value=w2
  Peak : Outport
  Fxmax : Outport  Port=2
  wires:
  1-a15*camber^2/1 -> ((a1Fz+a2)Fz) (1-a15*camber^2)/2
  const=1_2/1 -> 1-a15*camber^2/1
  const=2_2/1 -> camber^2/2
  a1Fz/1 -> a1Fz+a2/1
  camber/1 -> camber^2/1
  a15*camber^2/1 -> 1-a15*camber^2/2
  (a1Fz+a2)Fz/1 -> ((a1Fz+a2)Fz) (1-a15*camber^2)/1
  a15/1 -> a15*camber^2/1
  camber^2/1 -> a15*camber^2/2
  a1Fz+a2/1 -> (a1Fz+a2)Fz/2
  [Fz] -> a1Fz/1, (a1Fz+a2)Fz/1
  a1/1 -> a1Fz/2
  a2/1 -> a1Fz+a2/2
  "F_ymax* sqrt(1-(Fx*Fymax^-1)^2) "/1 -> abs(F_ymax* sqrt(1-(Fx*Fymax^-1)^2) )/1
  [F_ymax] -> "F_ymax* sqrt(1-(Fx*Fymax^-1)^2) "/1
  sqrt(1-(Fx*Fymax^-1)^2)/1 -> "F_ymax* sqrt(1-(Fx*Fymax^-1)^2) "/2
  const=1/1 -> 1-(Fx*Fymax^-1)^2/1
  1-(Fx*Fymax^-1)^2/1 -> sqrt(1-(Fx*Fymax^-1)^2)/1
  Fx/1 -> Fx*Fymax^-1/1
  Fx*Fymax^-1/1 -> (Fx*Fymax^-1)^2/1
  (Fx*Fymax^-1)^2/1 -> 1-(Fx*Fymax^-1)^2/2
  const=2/1 -> (Fx*Fymax^-1)^2/2
  [F_xmax] -> Fx*Fymax^-1/2
  (b1Fz+b2)Fz/1 -> D+V_long/1
  [Fz] -> b1Fz/1, (b1Fz+b2)Fz/1
  b1Fz+b2/1 -> (b1Fz+b2)Fz/2
  b1Fz/1 -> b1Fz+b2/1
  b2/1 -> b1Fz+b2/2
  b1/1 -> b1Fz/2
  b11/1 -> b11Fz/1
  b11Fz/1 -> b11Fz+b12/1
  [Fz] -> b11Fz/2
  b12/1 -> b11Fz+b12/2
  b11Fz+b12/1 -> D+V_long/2
  const=1_3/1 -> 1 ------ w1*wear+w2/1
  w1*wear+w2/1 -> 1 ------ w1*wear+w2/2
  w2/1 -> w1*wear+w2/2
  w1*wear/1 -> w1*wear+w2/1
  Wear/1 -> w1*wear/1
  1 ------ w1*wear+w2/1 -> (D+V_long)*wear/1, (D+V_lat)*wear/2
  (D+V_lat)*wear/1 -> [F_ymax]
  (D+V_long)*wear/1 -> [F_xmax]
  D+V_long/1 -> (D+V_long)*wear/2
  ((a1Fz+a2)Fz) (1-a15*camber^2)/1 -> D+V_lat/1
  D+V_lat/1 -> (D+V_lat)*wear/1
  a12/1 -> a13Fz+a14+Fz+camber +a12+a11Fz/2
  a13Fz+a14/1 -> a13Fz+a14+Fz+camber/1
  [Fz] -> a13Fz/2
  a14/1 -> a13Fz+a14/2
  a13Fz+a14+Fz+camber/1 -> a13Fz+a14+Fz+camber +a12+a11Fz/3
  a13/1 -> a13Fz/1
  a13Fz/1 -> a13Fz+a14/1
  Constant11/1 -> a13Fz+a14+Fz+camber/3
  a11/1 -> a11Fz/1
  a11Fz/1 -> a13Fz+a14+Fz+camber +a12+a11Fz/1
  [Fz] -> a11Fz/2
  [Fz] -> a13Fz+a14+Fz+camber/2
  Fz/1 -> Fz*10^-3/1
  Fz*10^-3/1 -> [Fz]
  a13Fz+a14+Fz+camber +a12+a11Fz/1 -> [V_lat]
  [V_lat] -> D+V_lat/2
  abs(F_ymax* sqrt(1-(Fx*Fymax^-1)^2) )/1 -> newD+V/1
  newD+V/1 -> Peak/1
  [V_lat] -> newD+V/2
  [F_xmax] -> Fxmax/1

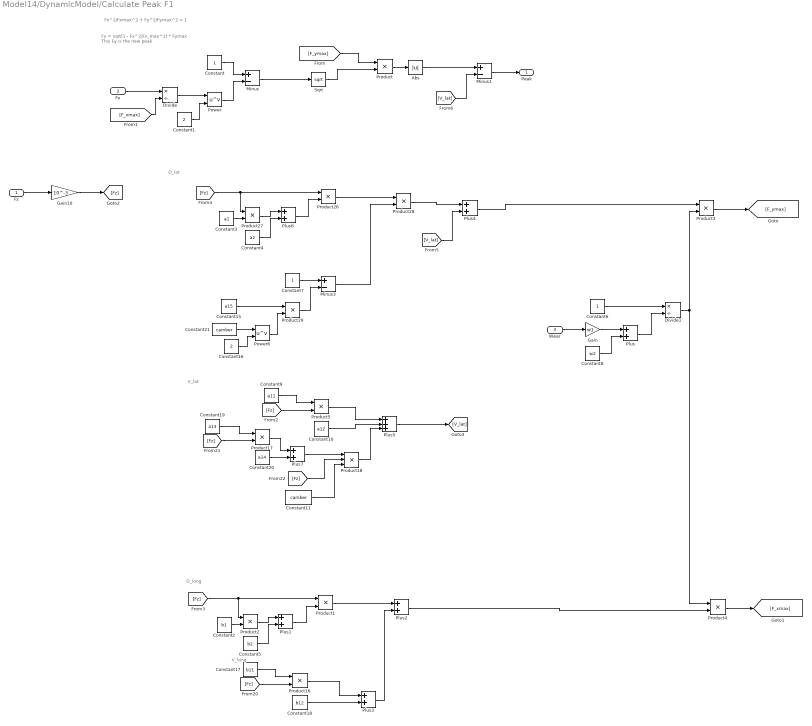
== system Model14/DynamicModel/Calculate Peak F1 ==
  note: V_lat
  note: D_lat
  note: D_long
  note: V_long
  note: Fy = sqrt(1 - Fx^2/Fx_max^2) * Fymax
      |
      | This Fy is the new peak
  note: Fx^2/Fxmax^2 + Fy^2/Fymax^2 = 1
  Fz : Inport  Unit=N
  Fx : Inport  Port=2  Unit=N
  Wear : Inport  Port=3
  Abs : Abs
  Constant : Constant
  Constant1 : Constant  Value=2
  Constant10 : Constant  Value=a12
  Constant11 : Constant  Value=camber
  Constant15 : Constant  Value=a15
  Constant16 : Constant  Value=2
  Constant17 : Constant  Value=b11
  Constant18 : Constant  Value=b12
  Constant19 : Constant  Value=a13
  Constant2 : Constant  Value=b1
  Constant20 : Constant  Value=a14
  Constant21 : Constant  Value=camber
  Constant3 : Constant  Value=a1
  Constant4 : Constant  Value=a2
  Constant5 : Constant  Value=b2
  Constant6 : Constant
  Constant7 : Constant
  Constant8 : Constant  Value=w2
  Constant9 : Constant  Value=a11
  Divide : Product  Inputs=*/
  Divide1 : Product  Inputs=*/
  Gain : Gain  Gain=w1
  Gain10 : Gain  Gain=10^-3
  Minus : Sum  Inputs=+-
  Minus1 : Sum  Inputs=+-
  Minus3 : Sum  Inputs=+-
  Plus{,1..4,6..7} (7 alike) : Sum
  Plus5 : Sum  Inputs=+++
  Power : Math  Operator=pow  SaturateOnIntegerOverflow=on
  Power6 : Math  Operator=pow  SaturateOnIntegerOverflow=on
  Product{,1..5,16..17,26..29} (12 alike) : Product
  Product18 : Product  Inputs=3
  Sqrt : Sqrt  SaturateOnIntegerOverflow=on
  Peak : Outport
  wires:
  Minus3/1 -> Product28/2
  Constant7/1 -> Minus3/1
  Constant16/1 -> Power6/2
  Product27/1 -> Plus6/1
  Constant21/1 -> Power6/1
  Product29/1 -> Minus3/2
  Product26/1 -> Product28/1
  Constant15/1 -> Product29/1
  Power6/1 -> Product29/2
  Plus6/1 -> Product26/2
  [Fz] -> Product27/1, Product26/1
  Constant3/1 -> Product27/2
  Constant4/1 -> Plus6/2
  Product/1 -> Abs/1
  [F_ymax] -> Product/1
  Sqrt/1 -> Product/2
  Constant/1 -> Minus/1
  Minus/1 -> Sqrt/1
  Fx/1 -> Divide/1
  Divide/1 -> Power/1
  Power/1 -> Minus/2
  Constant1/1 -> Power/2
  [F_xmax] -> Divide/2
  Product1/1 -> Plus2/1
  [Fz] -> Product2/1, Product1/1
  Plus1/1 -> Product1/2
  Product2/1 -> Plus1/1
  Constant5/1 -> Plus1/2
  Constant2/1 -> Product2/2
  Constant17/1 -> Product16/1
  Product16/1 -> Plus3/1
  [Fz] -> Product16/2
  Constant18/1 -> Plus3/2
  Plus3/1 -> Plus2/2
  Constant6/1 -> Divide1/1
  Plus/1 -> Divide1/2
  Constant8/1 -> Plus/2
  Gain/1 -> Plus/1
  Wear/1 -> Gain/1
  Divide1/1 -> Product4/1, Product3/2
  Product3/1 -> [F_ymax]
  Product4/1 -> [F_xmax]
  Plus2/1 -> Product4/2
  Product28/1 -> Plus4/1
  Plus4/1 -> Product3/1
  Constant10/1 -> Plus5/2
  Plus7/1 -> Product18/1
  [Fz] -> Product17/2
  Constant20/1 -> Plus7/2
  Product18/1 -> Plus5/3
  Constant19/1 -> Product17/1
  Product17/1 -> Plus7/1
  Constant11/1 -> Product18/3
  Constant9/1 -> Product5/1
  Product5/1 -> Plus5/1
  [Fz] -> Product5/2
  [Fz] -> Product18/2
  Fz/1 -> Gain10/1
  Gain10/1 -> [Fz]
  Plus5/1 -> [V_lat]
  [V_lat] -> Plus4/2
  Abs/1 -> Minus1/1
  Minus1/1 -> Peak/1
  [V_lat] -> Minus1/2

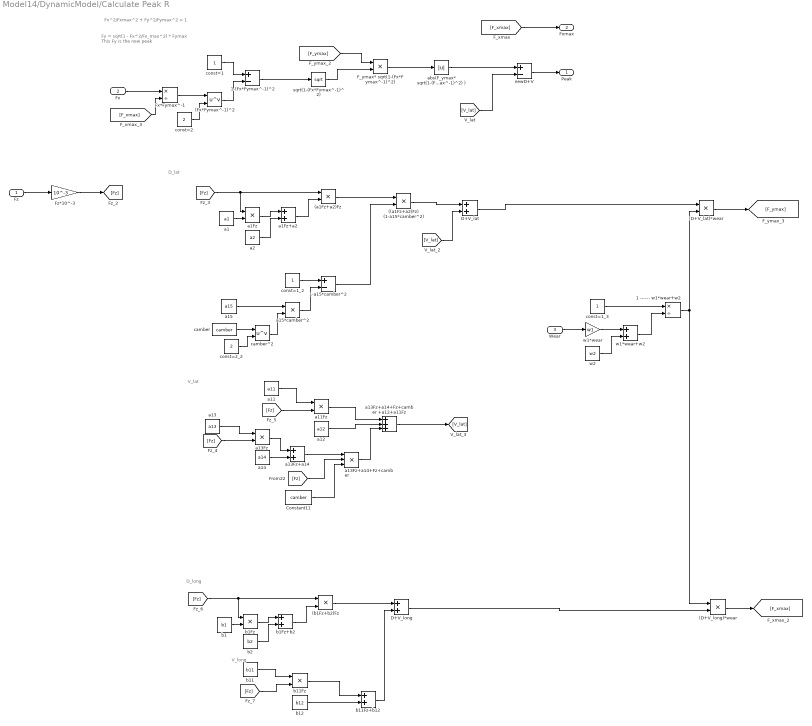
== system Model14/DynamicModel/Calculate Peak R ==
  note: V_lat
  note: D_lat
  note: D_long
  note: V_long
  note: Fy = sqrt(1 - Fx^2/Fx_max^2) * Fymax
      |
      | This Fy is the new peak
  note: Fx^2/Fxmax^2 + Fy^2/Fymax^2 = 1
  Fz : Inport  Unit=N
  Fx : Inport  Port=2  Unit=N
  Wear : Inport  Port=3
  ((a1Fz+a2)Fz) (1-a15*camber^2) : Product
  (D+V_lat)*wear : Product
  (D+V_long)*wear : Product
  (Fx*Fymax^-1)^2 : Math  Operator=pow  SaturateOnIntegerOverflow=on
  (a1Fz+a2)Fz : Product
  (b1Fz+b2)Fz : Product
  1 ------ w1*wear+w2 : Product  Inputs=*/
  1-(Fx*Fymax^-1)^2 : Sum  Inputs=+-
  1-a15*camber^2 : Sum  Inputs=+-
  Constant11 : Constant  Value=camber
  D+V_lat : Sum
  D+V_long : Sum
  "F_ymax* sqrt(1-(Fx*Fymax^-1)^2) " : Product
  Fx*Fymax^-1 : Product  Inputs=*/
  Fz*10^-3 : Gain  Gain=10^-3
  a1 : Constant  Value=a1
  a11 : Constant  Value=a11
  a11Fz : Product
  a12 : Constant  Value=a12
  a13 : Constant  Value=a13
  a13Fz : Product
  a13Fz+a14 : Sum
  a13Fz+a14+Fz+camber : Product  Inputs=3
  a13Fz+a14+Fz+camber +a12+a11Fz : Sum  Inputs=+++
  a14 : Constant  Value=a14
  a15 : Constant  Value=a15
  a15*camber^2 : Product
  a1Fz : Product
  a1Fz+a2 : Sum
  a2 : Constant  Value=a2
  abs(F_ymax* sqrt(1-(Fx*Fymax^-1)^2) ) : Abs
  b1 : Constant  Value=b1
  b11 : Constant  Value=b11
  b11Fz : Product
  b11Fz+b12 : Sum
  b12 : Constant  Value=b12
  b1Fz : Product
  b1Fz+b2 : Sum
  b2 : Constant  Value=b2
  camber : Constant  Value=camber
  camber^2 : Math  Operator=pow  SaturateOnIntegerOverflow=on
  const=1 : Constant
  const=1_2 : Constant
  const=1_3 : Constant
  const=2 : Constant  Value=2
  const=2_2 : Constant  Value=2
  newD+V : Sum  Inputs=+-
  sqrt(1-(Fx*Fymax^-1)^2) : Sqrt  SaturateOnIntegerOverflow=on
  w1*wear : Gain  Gain=w1
  w1*wear+w2 : Sum
  w2 : Constant  Value=w2
  Peak : Outport
  Fxmax : Outport  Port=2
  wires:
  1-a15*camber^2/1 -> ((a1Fz+a2)Fz) (1-a15*camber^2)/2
  const=1_2/1 -> 1-a15*camber^2/1
  const=2_2/1 -> camber^2/2
  a1Fz/1 -> a1Fz+a2/1
  camber/1 -> camber^2/1
  a15*camber^2/1 -> 1-a15*camber^2/2
  (a1Fz+a2)Fz/1 -> ((a1Fz+a2)Fz) (1-a15*camber^2)/1
  a15/1 -> a15*camber^2/1
  camber^2/1 -> a15*camber^2/2
  a1Fz+a2/1 -> (a1Fz+a2)Fz/2
  [Fz] -> a1Fz/1, (a1Fz+a2)Fz/1
  a1/1 -> a1Fz/2
  a2/1 -> a1Fz+a2/2
  "F_ymax* sqrt(1-(Fx*Fymax^-1)^2) "/1 -> abs(F_ymax* sqrt(1-(Fx*Fymax^-1)^2) )/1
  [F_ymax] -> "F_ymax* sqrt(1-(Fx*Fymax^-1)^2) "/1
  sqrt(1-(Fx*Fymax^-1)^2)/1 -> "F_ymax* sqrt(1-(Fx*Fymax^-1)^2) "/2
  const=1/1 -> 1-(Fx*Fymax^-1)^2/1
  1-(Fx*Fymax^-1)^2/1 -> sqrt(1-(Fx*Fymax^-1)^2)/1
  Fx/1 -> Fx*Fymax^-1/1
  Fx*Fymax^-1/1 -> (Fx*Fymax^-1)^2/1
  (Fx*Fymax^-1)^2/1 -> 1-(Fx*Fymax^-1)^2/2
  const=2/1 -> (Fx*Fymax^-1)^2/2
  [F_xmax] -> Fx*Fymax^-1/2
  (b1Fz+b2)Fz/1 -> D+V_long/1
  [Fz] -> b1Fz/1, (b1Fz+b2)Fz/1
  b1Fz+b2/1 -> (b1Fz+b2)Fz/2
  b1Fz/1 -> b1Fz+b2/1
  b2/1 -> b1Fz+b2/2
  b1/1 -> b1Fz/2
  b11/1 -> b11Fz/1
  b11Fz/1 -> b11Fz+b12/1
  [Fz] -> b11Fz/2
  b12/1 -> b11Fz+b12/2
  b11Fz+b12/1 -> D+V_long/2
  const=1_3/1 -> 1 ------ w1*wear+w2/1
  w1*wear+w2/1 -> 1 ------ w1*wear+w2/2
  w2/1 -> w1*wear+w2/2
  w1*wear/1 -> w1*wear+w2/1
  Wear/1 -> w1*wear/1
  1 ------ w1*wear+w2/1 -> (D+V_long)*wear/1, (D+V_lat)*wear/2
  (D+V_lat)*wear/1 -> [F_ymax]
  (D+V_long)*wear/1 -> [F_xmax]
  D+V_long/1 -> (D+V_long)*wear/2
  ((a1Fz+a2)Fz) (1-a15*camber^2)/1 -> D+V_lat/1
  D+V_lat/1 -> (D+V_lat)*wear/1
  a12/1 -> a13Fz+a14+Fz+camber +a12+a11Fz/2
  a13Fz+a14/1 -> a13Fz+a14+Fz+camber/1
  [Fz] -> a13Fz/2
  a14/1 -> a13Fz+a14/2
  a13Fz+a14+Fz+camber/1 -> a13Fz+a14+Fz+camber +a12+a11Fz/3
  a13/1 -> a13Fz/1
  a13Fz/1 -> a13Fz+a14/1
  Constant11/1 -> a13Fz+a14+Fz+camber/3
  a11/1 -> a11Fz/1
  a11Fz/1 -> a13Fz+a14+Fz+camber +a12+a11Fz/1
  [Fz] -> a11Fz/2
  [Fz] -> a13Fz+a14+Fz+camber/2
  Fz/1 -> Fz*10^-3/1
  Fz*10^-3/1 -> [Fz]
  a13Fz+a14+Fz+camber +a12+a11Fz/1 -> [V_lat]
  [V_lat] -> D+V_lat/2
  abs(F_ymax* sqrt(1-(Fx*Fymax^-1)^2) )/1 -> newD+V/1
  newD+V/1 -> Peak/1
  [V_lat] -> newD+V/2
  [F_xmax] -> Fxmax/1

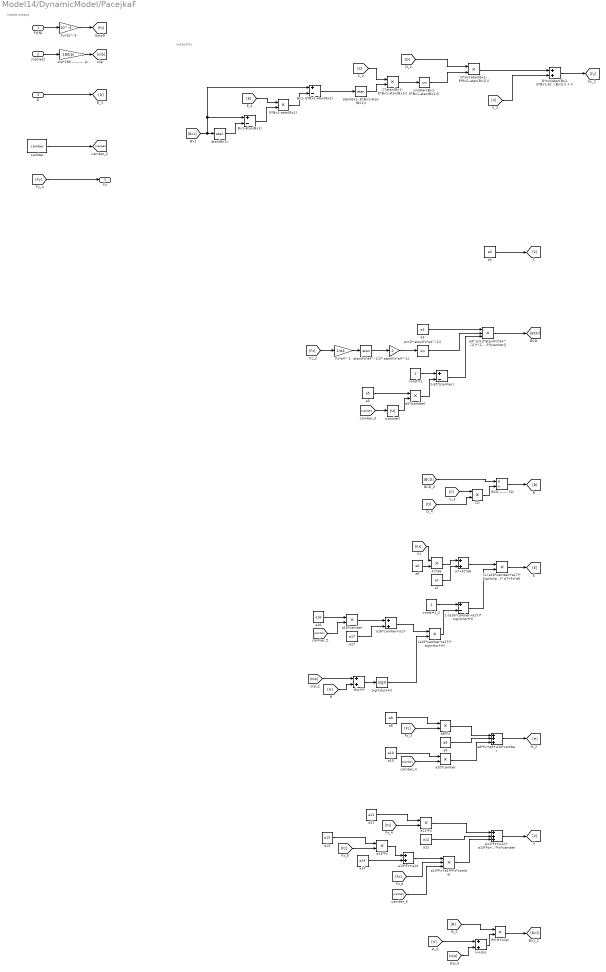
== system Model14/DynamicModel/PacejkaF ==
  note: inputs-output
  note: output-Fy
  Fz[N] : Inport  Unit=N
  slip[rad] : Inport  Port=2  Unit=rad
  D : Inport  Port=3
  (1-(a16*camber+a17)* sign(slip+H))* a7+Fz*a6 : Product
  (a16*camber+a17)* sign(slip+H) : Product
  1-(a16*camber+a17)* sign(slip+H) : Sum  Inputs=+-
  1-a5*|camber| : Sum  Inputs=+-
  2* atan(Fz*a4^-1) : Gain  Gain=2
  B*(H+slip) : Product
  BCD ------ CD : Product  Inputs=*/
  Bx1- E*Bx1-atan(Bx1) : Sum  Inputs=+-
  Bx1-atan(Bx1) : Sum  Inputs=+-
  C*atan(Bx1- E*Bx1-atan(Bx1)) : Product
  CD : Product
  D*sin(atan(Bx1- E*Bx1-atan(Bx1))) : Product
  D*sin(atan(Bx1- E*Bx1-atan(Bx1))) + V : Sum
  E*Bx1-atan(Bx1) : Product
  Fz*10^-3 : Gain  Gain=10^-3
  Fz*a4^-1 : Gain  Gain=1/a4
  Fz*a6 : Product
  H+slip : Sum
  a0 : Constant  Value=a0
  a10 : Constant  Value=a10
  a10*camber : Product
  a11 : Constant  Value=a11
  a11*Fz : Product
  a11*Fz+a12+ a13*Fz+a14*Fz*camber : Sum  Inputs=+++
  a12 : Constant  Value=a12
  a13 : Constant  Value=a13
  a13*Fz : Product
  a13*Fz+a14 : Sum
  a13*Fz+a14*Fz*camber : Product  Inputs=3
  a14 : Constant  Value=a14
  a16 : Constant  Value=a16
  a16*camber : Product
  a16*camber+a17 : Sum
  a17 : Constant  Value=a17
  a3 : Constant  Value=a3
  a3* sin(2*atan(Fz*a4^-1))* (1-a5*|camber|) : Product  Inputs=3
  a5 : Constant  Value=a5
  a5*|camber| : Product
  a6 : Constant  Value=a6
  a7 : Constant  Value=a7
  a7+Fz*a6 : Sum
  a8 : Constant  Value=a8
  a8*Fz : Product
  a8*Fz+a9+a10*camber : Sum  Inputs=+++
  a9 : Constant  Value=a9
  atan(Bx1) : Trigonometry  Operator=atan
  atan(Bx1- E*Bx1-atan(Bx1)) : Trigonometry  Operator=atan
  atan(Fz*a4^-1) : Trigonometry  Operator=atan
  camber : Constant  Value=camber
  const=1 : Constant
  const=1_2 : Constant
  sign(slip+H) : Signum  ZeroCross=off
  sin(2* atan(Fz*a4^-1)) : Trigonometry
  sin(atan(Bx1- E*Bx1-atan(Bx1))) : Trigonometry
  slip*180 --------- pi : Gain  Gain=180/pi
  slip+H : Sum
  |camber| : Abs
  Fy : Outport  Unit=N
  wires:
  C*atan(Bx1- E*Bx1-atan(Bx1))/1 -> sin(atan(Bx1- E*Bx1-atan(Bx1)))/1
  E*Bx1-atan(Bx1)/1 -> Bx1- E*Bx1-atan(Bx1)/2
  slip[rad]/1 -> slip*180 --------- pi/1
  1-a5*|camber|/1 -> a3* sin(2*atan(Fz*a4^-1))* (1-a5*|camber|)/3
  a10*camber/1 -> a8*Fz+a9+a10*camber/3
  |camber|/1 -> a5*|camber|/2
  a8/1 -> a8*Fz/1
  Fz*10^-3/1 -> [Fz]
  a0/1 -> [C]
  atan(Bx1- E*Bx1-atan(Bx1))/1 -> C*atan(Bx1- E*Bx1-atan(Bx1))/2
  [Fy] -> Fy/1
  Fz*a4^-1/1 -> atan(Fz*a4^-1)/1
  [B] -> B*(H+slip)/1
  [Fz] -> a8*Fz/2
  [Bx1] -> atan(Bx1)/1, Bx1-atan(Bx1)/1, Bx1- E*Bx1-atan(Bx1)/1
  [Fz] -> a13*Fz+a14*Fz*camber/2
  slip*180 --------- pi/1 -> [slip]
  2* atan(Fz*a4^-1)/1 -> sin(2* atan(Fz*a4^-1))/1
  [Fz] -> Fz*a6/1
  [slip] -> H+slip/2
  a11*Fz+a12+ a13*Fz+a14*Fz*camber/1 -> [V]
  a7+Fz*a6/1 -> (1-(a16*camber+a17)* sign(slip+H))* a7+Fz*a6/1
  [D] -> D*sin(atan(Bx1- E*Bx1-atan(Bx1)))/1
  a8*Fz+a9+a10*camber/1 -> [H]
  1-(a16*camber+a17)* sign(slip+H)/1 -> (1-(a16*camber+a17)* sign(slip+H))* a7+Fz*a6/2
  Bx1- E*Bx1-atan(Bx1)/1 -> atan(Bx1- E*Bx1-atan(Bx1))/1
  a3/1 -> a3* sin(2*atan(Fz*a4^-1))* (1-a5*|camber|)/1
  [camber] -> a16*camber/2
  [V] -> D*sin(atan(Bx1- E*Bx1-atan(Bx1))) + V/2
  [C] -> C*atan(Bx1- E*Bx1-atan(Bx1))/1
  B*(H+slip)/1 -> [Bx1]
  Fz[N]/1 -> Fz*10^-3/1
  camber/1 -> [camber]
  a11*Fz/1 -> a11*Fz+a12+ a13*Fz+a14*Fz*camber/1
  const=1/1 -> 1-a5*|camber|/1
  [Fz] -> a13*Fz/2
  a8*Fz/1 -> a8*Fz+a9+a10*camber/1
  [BCD] -> BCD ------ CD/1
  a14/1 -> a13*Fz+a14/2
  sin(atan(Bx1- E*Bx1-atan(Bx1)))/1 -> D*sin(atan(Bx1- E*Bx1-atan(Bx1)))/2
  sign(slip+H)/1 -> (a16*camber+a17)* sign(slip+H)/2
  a3* sin(2*atan(Fz*a4^-1))* (1-a5*|camber|)/1 -> [BCD]
  [camber] -> |camber|/1
  a13*Fz+a14/1 -> a13*Fz+a14*Fz*camber/1
  a9/1 -> a8*Fz+a9+a10*camber/2
  a16*camber/1 -> a16*camber+a17/1
  a12/1 -> a11*Fz+a12+ a13*Fz+a14*Fz*camber/2
  (1-(a16*camber+a17)* sign(slip+H))* a7+Fz*a6/1 -> [E]
  [Fz] -> Fz*a4^-1/1
  D*sin(atan(Bx1- E*Bx1-atan(Bx1))) + V/1 -> [Fy]
  BCD ------ CD/1 -> [B]
  a10/1 -> a10*camber/1
  [H] -> H+slip/1
  atan(Fz*a4^-1)/1 -> 2* atan(Fz*a4^-1)/1
  a16*camber+a17/1 -> (a16*camber+a17)* sign(slip+H)/1
  a11/1 -> a11*Fz/1
  a13*Fz/1 -> a13*Fz+a14/1
  a13*Fz+a14*Fz*camber/1 -> a11*Fz+a12+ a13*Fz+a14*Fz*camber/3
  a17/1 -> a16*camber+a17/2
  Fz*a6/1 -> a7+Fz*a6/1
  sin(2* atan(Fz*a4^-1))/1 -> a3* sin(2*atan(Fz*a4^-1))* (1-a5*|camber|)/2
  [Fz] -> a11*Fz/2
  [camber] -> a13*Fz+a14*Fz*camber/3
  Bx1-atan(Bx1)/1 -> E*Bx1-atan(Bx1)/2
  [C] -> CD/1
  [camber] -> a10*camber/2
  a6/1 -> Fz*a6/2
  [D] -> CD/2
  atan(Bx1)/1 -> Bx1-atan(Bx1)/2
  a13/1 -> a13*Fz/1
  (a16*camber+a17)* sign(slip+H)/1 -> 1-(a16*camber+a17)* sign(slip+H)/2
  D*sin(atan(Bx1- E*Bx1-atan(Bx1)))/1 -> D*sin(atan(Bx1- E*Bx1-atan(Bx1))) + V/1
  D/1 -> [D]
  H+slip/1 -> B*(H+slip)/2
  [E] -> E*Bx1-atan(Bx1)/1
  const=1_2/1 -> 1-(a16*camber+a17)* sign(slip+H)/1
  a7/1 -> a7+Fz*a6/2
  a16/1 -> a16*camber/1
  a5*|camber|/1 -> 1-a5*|camber|/2
  a5/1 -> a5*|camber|/1
  CD/1 -> BCD ------ CD/2
  [H] -> slip+H/2
  slip+H/1 -> sign(slip+H)/1
  [slip] -> slip+H/1

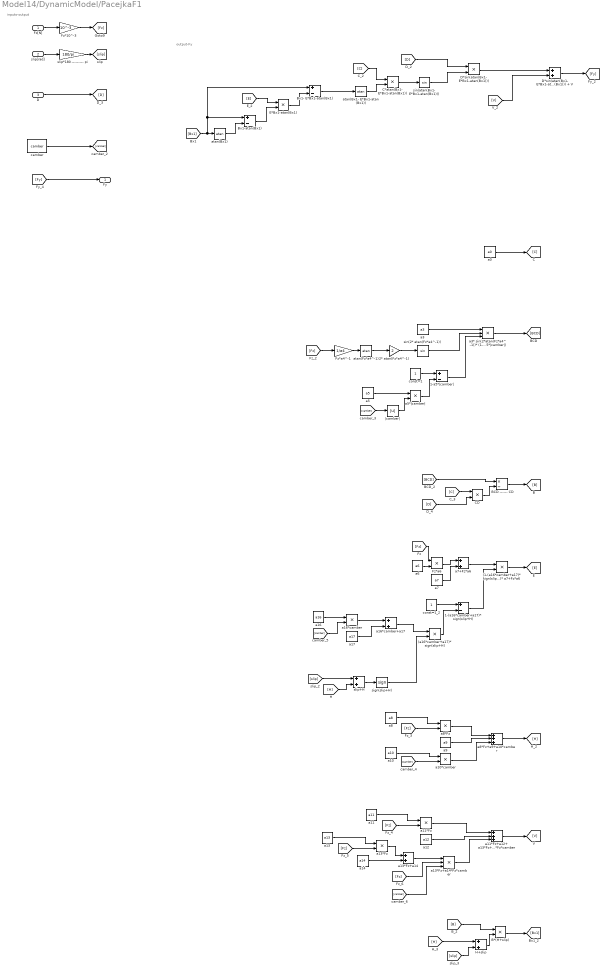
== system Model14/DynamicModel/PacejkaF1 ==
  note: inputs-output
  note: output-Fy
  Fz[N] : Inport  Unit=N
  slip[rad] : Inport  Port=2  Unit=rad
  D : Inport  Port=3
  (1-(a16*camber+a17)* sign(slip+H))* a7+Fz*a6 : Product
  (a16*camber+a17)* sign(slip+H) : Product
  1-(a16*camber+a17)* sign(slip+H) : Sum  Inputs=+-
  1-a5*|camber| : Sum  Inputs=+-
  2* atan(Fz*a4^-1) : Gain  Gain=2
  B*(H+slip) : Product
  BCD ------ CD : Product  Inputs=*/
  Bx1- E*Bx1-atan(Bx1) : Sum  Inputs=+-
  Bx1-atan(Bx1) : Sum  Inputs=+-
  C*atan(Bx1- E*Bx1-atan(Bx1)) : Product
  CD : Product
  D*sin(atan(Bx1- E*Bx1-atan(Bx1))) : Product
  D*sin(atan(Bx1- E*Bx1-atan(Bx1))) + V : Sum
  E*Bx1-atan(Bx1) : Product
  Fz*10^-3 : Gain  Gain=10^-3
  Fz*a4^-1 : Gain  Gain=1/a4
  Fz*a6 : Product
  H+slip : Sum
  a0 : Constant  Value=a0
  a10 : Constant  Value=a10
  a10*camber : Product
  a11 : Constant  Value=a11
  a11*Fz : Product
  a11*Fz+a12+ a13*Fz+a14*Fz*camber : Sum  Inputs=+++
  a12 : Constant  Value=a12
  a13 : Constant  Value=a13
  a13*Fz : Product
  a13*Fz+a14 : Sum
  a13*Fz+a14*Fz*camber : Product  Inputs=3
  a14 : Constant  Value=a14
  a16 : Constant  Value=a16
  a16*camber : Product
  a16*camber+a17 : Sum
  a17 : Constant  Value=a17
  a3 : Constant  Value=a3
  a3* sin(2*atan(Fz*a4^-1))* (1-a5*|camber|) : Product  Inputs=3
  a5 : Constant  Value=a5
  a5*|camber| : Product
  a6 : Constant  Value=a6
  a7 : Constant  Value=a7
  a7+Fz*a6 : Sum
  a8 : Constant  Value=a8
  a8*Fz : Product
  a8*Fz+a9+a10*camber : Sum  Inputs=+++
  a9 : Constant  Value=a9
  atan(Bx1) : Trigonometry  Operator=atan
  atan(Bx1- E*Bx1-atan(Bx1)) : Trigonometry  Operator=atan
  atan(Fz*a4^-1) : Trigonometry  Operator=atan
  camber : Constant  Value=camber
  const=1 : Constant
  const=1_2 : Constant
  sign(slip+H) : Signum  ZeroCross=off
  sin(2* atan(Fz*a4^-1)) : Trigonometry
  sin(atan(Bx1- E*Bx1-atan(Bx1))) : Trigonometry
  slip*180 --------- pi : Gain  Gain=180/pi
  slip+H : Sum
  |camber| : Abs
  Fy : Outport  Unit=N
  wires:
  C*atan(Bx1- E*Bx1-atan(Bx1))/1 -> sin(atan(Bx1- E*Bx1-atan(Bx1)))/1
  E*Bx1-atan(Bx1)/1 -> Bx1- E*Bx1-atan(Bx1)/2
  slip[rad]/1 -> slip*180 --------- pi/1
  1-a5*|camber|/1 -> a3* sin(2*atan(Fz*a4^-1))* (1-a5*|camber|)/3
  a10*camber/1 -> a8*Fz+a9+a10*camber/3
  |camber|/1 -> a5*|camber|/2
  a8/1 -> a8*Fz/1
  Fz*10^-3/1 -> [Fz]
  a0/1 -> [C]
  atan(Bx1- E*Bx1-atan(Bx1))/1 -> C*atan(Bx1- E*Bx1-atan(Bx1))/2
  [Fy] -> Fy/1
  Fz*a4^-1/1 -> atan(Fz*a4^-1)/1
  [B] -> B*(H+slip)/1
  [Fz] -> a8*Fz/2
  [Bx1] -> atan(Bx1)/1, Bx1-atan(Bx1)/1, Bx1- E*Bx1-atan(Bx1)/1
  [Fz] -> a13*Fz+a14*Fz*camber/2
  slip*180 --------- pi/1 -> [slip]
  2* atan(Fz*a4^-1)/1 -> sin(2* atan(Fz*a4^-1))/1
  [Fz] -> Fz*a6/1
  [slip] -> H+slip/2
  a11*Fz+a12+ a13*Fz+a14*Fz*camber/1 -> [V]
  a7+Fz*a6/1 -> (1-(a16*camber+a17)* sign(slip+H))* a7+Fz*a6/1
  [D] -> D*sin(atan(Bx1- E*Bx1-atan(Bx1)))/1
  a8*Fz+a9+a10*camber/1 -> [H]
  1-(a16*camber+a17)* sign(slip+H)/1 -> (1-(a16*camber+a17)* sign(slip+H))* a7+Fz*a6/2
  Bx1- E*Bx1-atan(Bx1)/1 -> atan(Bx1- E*Bx1-atan(Bx1))/1
  a3/1 -> a3* sin(2*atan(Fz*a4^-1))* (1-a5*|camber|)/1
  [camber] -> a16*camber/2
  [V] -> D*sin(atan(Bx1- E*Bx1-atan(Bx1))) + V/2
  [C] -> C*atan(Bx1- E*Bx1-atan(Bx1))/1
  B*(H+slip)/1 -> [Bx1]
  Fz[N]/1 -> Fz*10^-3/1
  camber/1 -> [camber]
  a11*Fz/1 -> a11*Fz+a12+ a13*Fz+a14*Fz*camber/1
  const=1/1 -> 1-a5*|camber|/1
  [Fz] -> a13*Fz/2
  a8*Fz/1 -> a8*Fz+a9+a10*camber/1
  [BCD] -> BCD ------ CD/1
  a14/1 -> a13*Fz+a14/2
  sin(atan(Bx1- E*Bx1-atan(Bx1)))/1 -> D*sin(atan(Bx1- E*Bx1-atan(Bx1)))/2
  sign(slip+H)/1 -> (a16*camber+a17)* sign(slip+H)/2
  a3* sin(2*atan(Fz*a4^-1))* (1-a5*|camber|)/1 -> [BCD]
  [camber] -> |camber|/1
  a13*Fz+a14/1 -> a13*Fz+a14*Fz*camber/1
  a9/1 -> a8*Fz+a9+a10*camber/2
  a16*camber/1 -> a16*camber+a17/1
  a12/1 -> a11*Fz+a12+ a13*Fz+a14*Fz*camber/2
  (1-(a16*camber+a17)* sign(slip+H))* a7+Fz*a6/1 -> [E]
  [Fz] -> Fz*a4^-1/1
  D*sin(atan(Bx1- E*Bx1-atan(Bx1))) + V/1 -> [Fy]
  BCD ------ CD/1 -> [B]
  a10/1 -> a10*camber/1
  [H] -> H+slip/1
  atan(Fz*a4^-1)/1 -> 2* atan(Fz*a4^-1)/1
  a16*camber+a17/1 -> (a16*camber+a17)* sign(slip+H)/1
  a11/1 -> a11*Fz/1
  a13*Fz/1 -> a13*Fz+a14/1
  a13*Fz+a14*Fz*camber/1 -> a11*Fz+a12+ a13*Fz+a14*Fz*camber/3
  a17/1 -> a16*camber+a17/2
  Fz*a6/1 -> a7+Fz*a6/1
  sin(2* atan(Fz*a4^-1))/1 -> a3* sin(2*atan(Fz*a4^-1))* (1-a5*|camber|)/2
  [Fz] -> a11*Fz/2
  [camber] -> a13*Fz+a14*Fz*camber/3
  Bx1-atan(Bx1)/1 -> E*Bx1-atan(Bx1)/2
  [C] -> CD/1
  [camber] -> a10*camber/2
  a6/1 -> Fz*a6/2
  [D] -> CD/2
  atan(Bx1)/1 -> Bx1-atan(Bx1)/2
  a13/1 -> a13*Fz/1
  (a16*camber+a17)* sign(slip+H)/1 -> 1-(a16*camber+a17)* sign(slip+H)/2
  D*sin(atan(Bx1- E*Bx1-atan(Bx1)))/1 -> D*sin(atan(Bx1- E*Bx1-atan(Bx1))) + V/1
  D/1 -> [D]
  H+slip/1 -> B*(H+slip)/2
  [E] -> E*Bx1-atan(Bx1)/1
  const=1_2/1 -> 1-(a16*camber+a17)* sign(slip+H)/1
  a7/1 -> a7+Fz*a6/2
  a16/1 -> a16*camber/1
  a5*|camber|/1 -> 1-a5*|camber|/2
  a5/1 -> a5*|camber|/1
  CD/1 -> BCD ------ CD/2
  [H] -> slip+H/2
  slip+H/1 -> sign(slip+H)/1
  [slip] -> slip+H/1
